simulink model "UDE"  (R2019b)
settings: Solver=ode4  StartTime=0.0  StopTime=tstop  FixedStep=tstep  RelTol=1e-3
values from neighbouring files (symbols this model uses):
  Ts = 0.01    [data.m]
  xic = [-3 2]'    [data.m]
settings Model: Creator=Ram Padmanabhan  LastModifiedBy=Maithili Shetty
settings DataIOCC: SaveOutput=off  SignalLogging=off  DSMLogging=off  SaveTime=off  ReturnWorkspaceOutputs=off

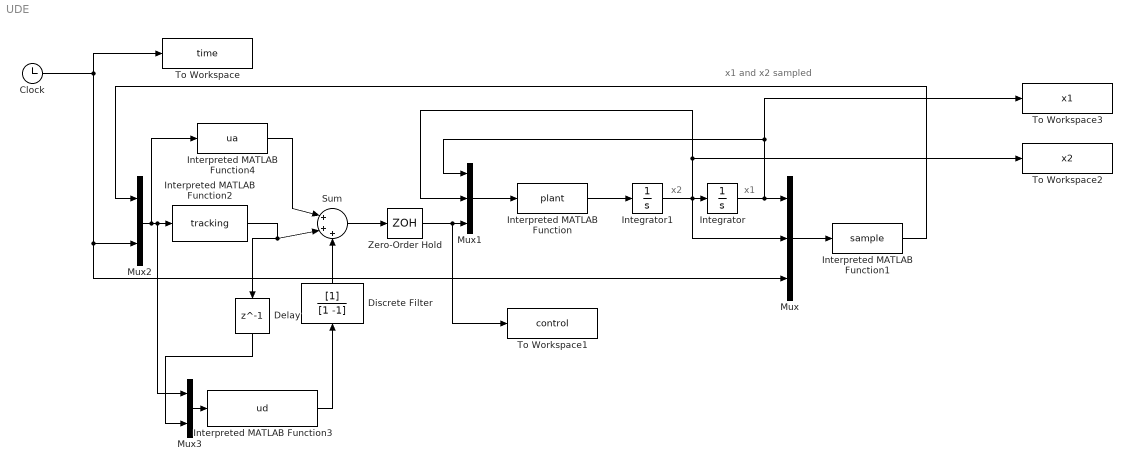
== system UDE ==
  note: x1 and x2 sampled
  note: x1
  note: x2
  Clock : Clock
  Delay : Delay  DelayLength=1  InitialCondition=0  SampleTime=Ts
  Discrete Filter : DiscreteFilter  Denominator=[1 -1]  SampleTime=Ts
  Integrator : Integrator  InitialCondition=xic(1)
  Integrator1 : Integrator  InitialCondition=xic(2)
  Interpreted MATLAB Function : MATLABFcn  MATLABFcn=plant  OutputDimensions=1
  Interpreted MATLAB Function1 : MATLABFcn  MATLABFcn=sample  OutputDimensions=2
  Interpreted MATLAB Function2 : MATLABFcn  MATLABFcn=tracking  OutputDimensions=1
  Interpreted MATLAB Function3 : MATLABFcn  MATLABFcn=ud  OutputDimensions=1
  Interpreted MATLAB Function4 : MATLABFcn  MATLABFcn=ua  OutputDimensions=1
  Mux : Mux  Inputs=3
  Mux1 : Mux  Inputs=3
  Mux2 : Mux  Inputs=2
  Mux3 : Mux  Inputs=2
  Sum : Sum  Inputs=|+++
  To Workspace : ToWorkspace  VariableName=time  SampleTime=-1
  To Workspace1 : ToWorkspace  VariableName=control  SampleTime=-1
  To Workspace2 : ToWorkspace  VariableName=x2  SampleTime=-1
  To Workspace3 : ToWorkspace  VariableName=x1  SampleTime=-1
  Zero-Order Hold : ZeroOrderHold  SampleTime=Ts
  wires:
  Integrator1/1 -> Mux/2, Mux1/2, To Workspace2/1, Integrator/1
  Interpreted MATLAB Function/1 -> Integrator1/1
  Integrator/1 -> To Workspace3/1, Mux1/1, Mux/1
  Mux/1 -> Interpreted MATLAB Function1/1
  Clock/1 -> To Workspace/1, Mux2/2, Mux/3
  Mux1/1 -> Interpreted MATLAB Function/1
  Interpreted MATLAB Function2/1 -> Sum/2, Delay/1
  Interpreted MATLAB Function1/1 -> Mux2/1
  Mux2/1 -> Interpreted MATLAB Function4/1, Mux3/1, Interpreted MATLAB Function2/1
  Interpreted MATLAB Function3/1 -> Discrete Filter/1
  Zero-Order Hold/1 -> To Workspace1/1, Mux1/3
  Sum/1 -> Zero-Order Hold/1
  Mux3/1 -> Interpreted MATLAB Function3/1
  Delay/1 -> Mux3/2
  Discrete Filter/1 -> Sum/3
  Interpreted MATLAB Function4/1 -> Sum/1
